simulink model "om_M4"  (R2016a)
settings: Solver=FixedStepAuto  StartTime=0.0  StopTime=10  FixedStep=0.0005  RelTol=1e-3
values from neighbouring files (symbols this model uses):
  Lm = 0.1271    [motor4_workspace.mat]    (also in motor_wrapper.m = obj.Lm; scim_verifier.m = obj.motor.getLm(); setMotorParams.m; stationary_class.m = obj.Lm)
  Lr = 0.2744    [motor4_workspace.mat]    (also in motor_wrapper.m = obj.Lr; scim_verifier.m = obj.motor.getLr(); setMotorParams.m; stationary_class.m = obj.Lr)
  Ls = 0.2744    [motor4_workspace.mat]    (also in motor_wrapper.m = obj.Ls; scim_verifier.m = obj.motor.getLs(); setMotorParams.m; stationary.m = Ls/10)
  M_ab02abc = [1  0  1; -0.5  0.866025403784  1; -0.5  -0.866025403784  1]    [motor4_workspace.mat]    (also in setMotorParams.m = inv(M_abc2ab0); workspaceSav.mat)
  M_abc2ab0 = [0.666666666667  -0.333333333333  -0.333333333333; 0  0.57735026919  -0.57735026919; 0.333333333333  0.333333333333  0.333333333333]    [motor4_workspace.mat]    (also in setMotorParams.m = [1, -0.5, -0.5; 0, sqrt(3)/2, -sqrt(3)/2;  0.5, 0.5, 0.5]; workspaceSav.mat)
  Rr = 1.009    [motor4_workspace.mat]    (also in motor_wrapper.m = obj.Rr; setMotorParams.m; stationary_class.m = obj.Rr; stationary_from_eq.m = obj.Rr)
  sig = (tox-fromx)/6    [gaussSpace.m]    (also in motor4_workspace.mat = 0.785452782217; setMotorParams.m = 0.785452782217; stationary_class.m = 1-Lm*Lm/Ls/Lr; torqueFinder.m = 0.785452782217)
libraries: powerlib_meascontrol x2, simulink x1, simulink_extras x1
settings Model: Creator=ebenera  LastModifiedBy=ebenera

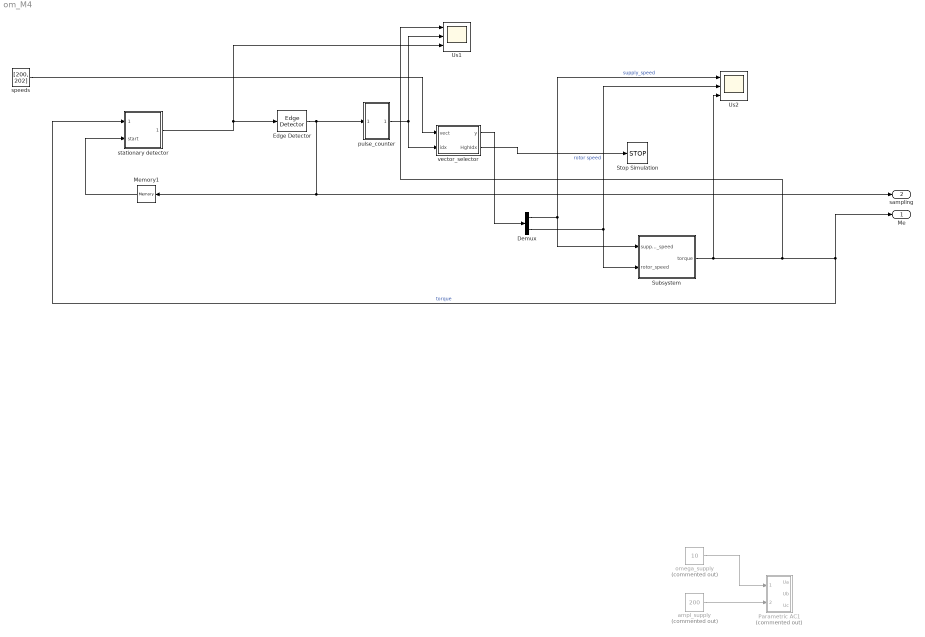
== system om_M4 ==
  Demux : Demux  Outputs=2
  Edge Detector : powerlib_meascontrol/Logic/Edge Detector  model=Rising  ic=0  Ts=0
  Memory1 : Memory  X0=1
  Parametric AC1 : Subsystem  Commented=on
  Stop Simulation : Stop
  Subsystem : Subsystem
  Us1 : Scope  NumInputPorts=3
  Us2 : Scope  NumInputPorts=3
  ampl_supply : Constant  Commented=on  Value=200
  omega_supply : Constant  Commented=on  Value=10
  pulse_counter : Subsystem
  speeds : Constant  Value=[200, 202]
  stationary detector : Subsystem
  vector_selector : MATLAB Function  TreatAsAtomicUnit=on
  Me : Outport
  sampling : Outport  Port=2
  wires:
  ampl_supply/1 -> Parametric AC1/2(Amp)
  omega_supply/1 -> Parametric AC1/1(Omega)
  speeds/1 -> vector_selector/1(vect)
  stationary detector/1(stable) -> Us1/3, Edge Detector/1
  vector_selector/2(HghIdx) -> Stop Simulation/1
  Subsystem/1(torque) -> Us2/3, Us1/1, stationary detector/1(state_var), Me/1  "torque"
  vector_selector/1(y) -> Demux/1
  Demux/2 -> Subsystem/2(rotor_speed), Us2/2  "rotor speed"
  Memory1/1 -> stationary detector/2(start)
  pulse_counter/1(Out1) -> vector_selector/2(idx), Us1/2
  Edge Detector/1 -> sampling/1, Memory1/1, pulse_counter/1(In1)
  Demux/1 -> Subsystem/1(supply_speed), Us2/1  "supply_speed"

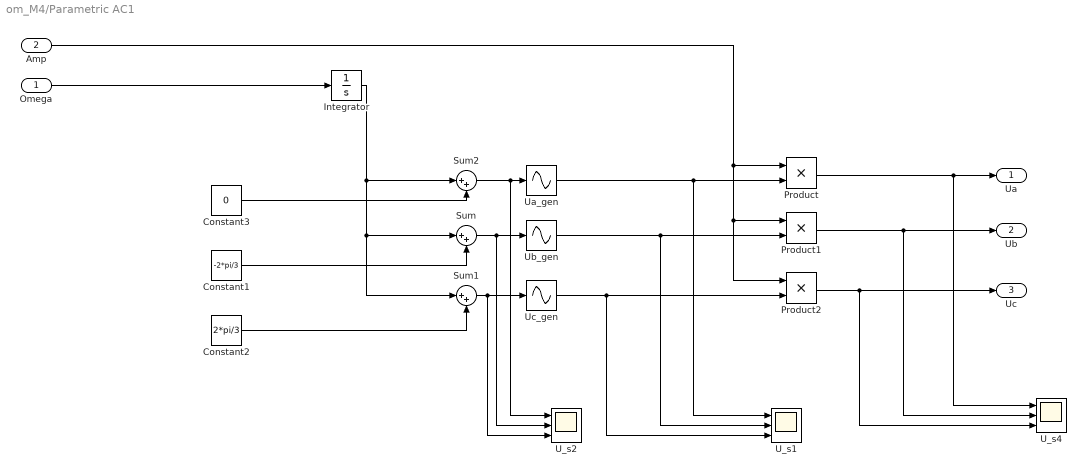
== system om_M4/Parametric AC1 ==
  Omega : Inport
  Amp : Inport  Port=2
  Constant1 : Constant  Value=-2*pi/3
  Constant2 : Constant  Value=2*pi/3
  Constant3 : Constant  Value=0
  Integrator : Integrator  WrapState=on
  Product : Product
  Product1 : Product
  Product2 : Product
  Sum : Sum  Inputs=|++
  Sum1 : Sum  Inputs=|++
  Sum2 : Sum  Inputs=|++
  U_s1 : Scope  NumInputPorts=3
  U_s2 : Scope  NumInputPorts=3
  U_s4 : Scope  NumInputPorts=3
  Ua_gen : Sin  TimeSource=Use external signal  SampleTime=0
  Ub_gen : Sin  TimeSource=Use external signal  SampleTime=0
  Uc_gen : Sin  TimeSource=Use external signal  SampleTime=0
  Ua : Outport
  Ub : Outport  Port=2
  Uc : Outport  Port=3
  wires:
  Sum/1 -> U_s2/2, Ub_gen/1
  Omega/1 -> Integrator/1
  Constant1/1 -> Sum/2
  Constant2/1 -> Sum1/2
  Sum1/1 -> U_s2/3, Uc_gen/1
  Sum2/1 -> U_s2/1, Ua_gen/1
  Constant3/1 -> Sum2/2
  Integrator/1 -> Sum2/1, Sum1/1, Sum/1
  Product/1 -> U_s4/1, Ua/1
  Product2/1 -> U_s4/3, Uc/1
  Product1/1 -> U_s4/2, Ub/1
  Amp/1 -> Product/1, Product1/1, Product2/1
  Ua_gen/1 -> U_s1/1, Product/2
  Uc_gen/1 -> U_s1/3, Product2/2
  Ub_gen/1 -> U_s1/2, Product1/2

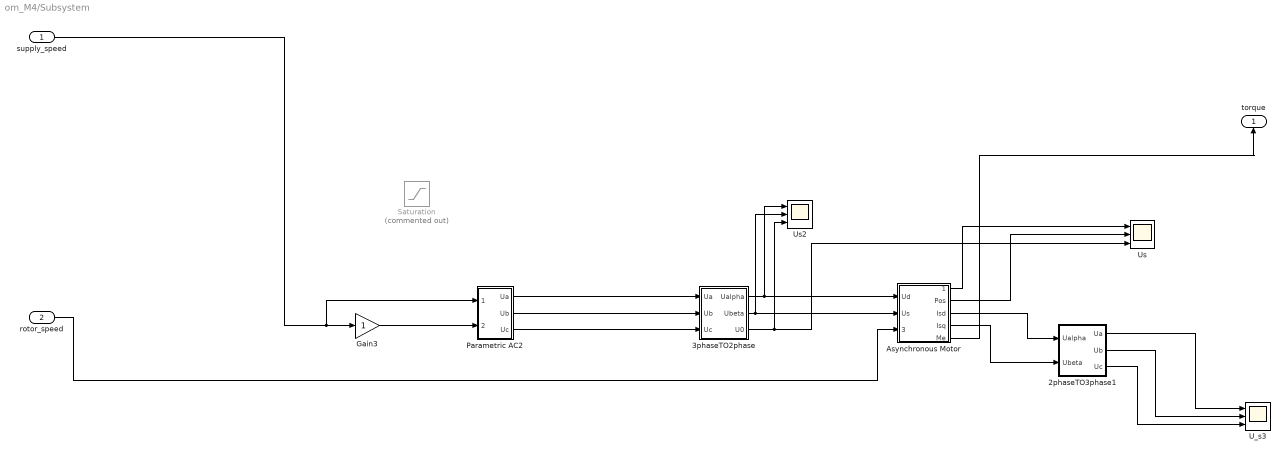
== system om_M4/Subsystem ==
  supply_speed : Inport
  rotor_speed : Inport  Port=2
  2phaseTO3phase1 : Subsystem
  "3phaseTO2phase " : Subsystem
  Asynchronous Motor : Subsystem
  Gain3 : Gain
  Parametric AC2 : Subsystem
  Saturation : Saturate  Commented=on  UpperLimit=300  LowerLimit=50
  U_s3 : Scope  NumInputPorts=3
  Us : Scope  NumInputPorts=3
  Us2 : Scope  NumInputPorts=3
  torque : Outport
  wires:
  "3phaseTO2phase "/1(Ualpha) -> Us2/1, Asynchronous Motor/1(Ud)
  "3phaseTO2phase "/2(Ubeta) -> Asynchronous Motor/2(Us), Us2/2
  Asynchronous Motor/4(Isq) -> 2phaseTO3phase1/2(Ubeta)
  Asynchronous Motor/3(Isd) -> 2phaseTO3phase1/1(Ualpha)
  2phaseTO3phase1/1(Ua) -> U_s3/1
  2phaseTO3phase1/2(Ub) -> U_s3/2
  2phaseTO3phase1/3(Uc) -> U_s3/3
  Parametric AC2/1(Ua) -> "3phaseTO2phase "/1(Ua)
  Parametric AC2/2(Ub) -> "3phaseTO2phase "/2(Ub)
  Parametric AC2/3(Uc) -> "3phaseTO2phase "/3(Uc)
  rotor_speed/1 -> Asynchronous Motor/3(OmegaIn)
  Asynchronous Motor/5(Me) -> torque/1
  Asynchronous Motor/1(Omega) -> Us/1
  Asynchronous Motor/2(Pos) -> Us/2
  "3phaseTO2phase "/3(U0) -> Us2/3, Us/3
  supply_speed/1 -> Gain3/1, Parametric AC2/1(Omega)
  Gain3/1 -> Parametric AC2/2(Amp)

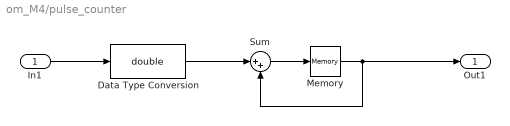
== system om_M4/pulse_counter ==
  In1 : Inport
  Data Type Conversion : DataTypeConversion  OutDataTypeStr=double  RndMeth=Ceiling
  Memory : Memory  X0=1
  Sum : Sum  Inputs=|++
  Out1 : Outport
  wires:
  Sum/1 -> Memory/1
  Memory/1 -> Sum/2, Out1/1
  In1/1 -> Data Type Conversion/1
  Data Type Conversion/1 -> Sum/1

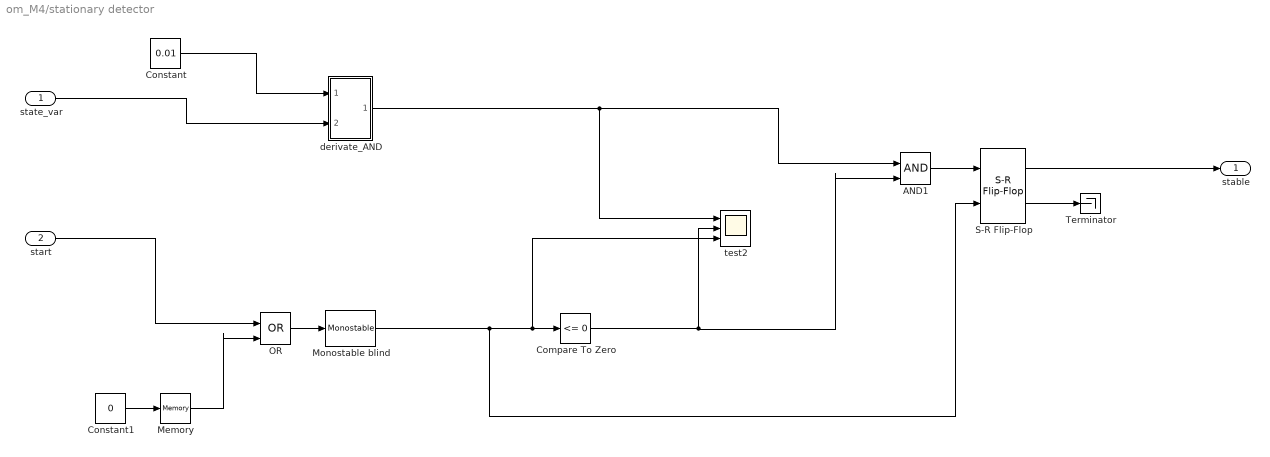
== system om_M4/stationary detector ==
  state_var : Inport
  start : Inport  Port=2
  AND1 : Logic  IconShape=distinctive  AllPortsSameDT=off  OutDataTypeStr=boolean
  Compare To Zero : simulink/Logic and Bit Operations/Compare To Zero  relop=<=  OutDataTypeStr=boolean
  Constant : Constant  Value=0.01
  Constant1 : Constant  Value=0
  Memory : Memory  X0=1
  Monostable blind : powerlib_meascontrol/Logic/Monostable  EdgeDetect=Either  PulseDuration=0.1  ic=0  Ts=0
  OR : Logic  Operator=OR  IconShape=distinctive  AllPortsSameDT=off  OutDataTypeStr=boolean
  S-R Flip-Flop : simulink_extras/Flip Flops/S-R Flip-Flop  initial_condition=0
  Terminator : Terminator
  derivate_AND : Subsystem
  test2 : Scope  NumInputPorts=3
  stable : Outport
  wires:
  Compare To Zero/1 -> AND1/2, test2/2
  S-R Flip-Flop/1 -> stable/1
  AND1/1 -> S-R Flip-Flop/1
  derivate_AND/1(Out1) -> AND1/1, test2/1
  Constant/1 -> derivate_AND/1(In1)
  state_var/1 -> derivate_AND/2(In2)
  Monostable blind/1 -> S-R Flip-Flop/2, test2/3, Compare To Zero/1
  Constant1/1 -> Memory/1
  Memory/1 -> OR/2
  start/1 -> OR/1
  OR/1 -> Monostable blind/1
  S-R Flip-Flop/2 -> Terminator/1

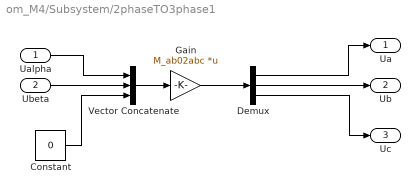
== system om_M4/Subsystem/2phaseTO3phase1 ==
  Ualpha : Inport
  Ubeta : Inport  Port=2
  Constant : Constant  Value=0
  Demux : Demux  Outputs=3
  Gain : Gain  Gain=M_ab02abc  Multiplication=Matrix(K*u)
  Vector Concatenate : Concatenate  NumInputs=3
  Ua : Outport
  Ub : Outport  Port=2
  Uc : Outport  Port=3
  wires:
  Vector Concatenate/1 -> Gain/1
  Ualpha/1 -> Vector Concatenate/1
  Demux/3 -> Uc/1
  Gain/1 -> Demux/1
  Constant/1 -> Vector Concatenate/3
  Ubeta/1 -> Vector Concatenate/2
  Demux/1 -> Ua/1
  Demux/2 -> Ub/1

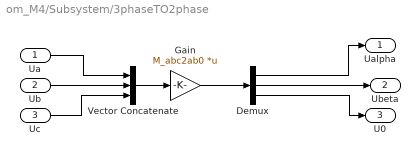
== system om_M4/Subsystem/3phaseTO2phase  ==
  Ua : Inport
  Ub : Inport  Port=2
  Uc : Inport  Port=3
  Demux : Demux  Outputs=3
  Gain : Gain  Gain=M_abc2ab0  Multiplication=Matrix(K*u)
  Vector Concatenate : Concatenate  NumInputs=3
  Ualpha : Outport
  Ubeta : Outport  Port=2
  U0 : Outport  Port=3
  wires:
  Vector Concatenate/1 -> Gain/1
  Ua/1 -> Vector Concatenate/1
  Demux/3 -> U0/1
  Gain/1 -> Demux/1
  Uc/1 -> Vector Concatenate/3
  Ub/1 -> Vector Concatenate/2
  Demux/1 -> Ualpha/1
  Demux/2 -> Ubeta/1

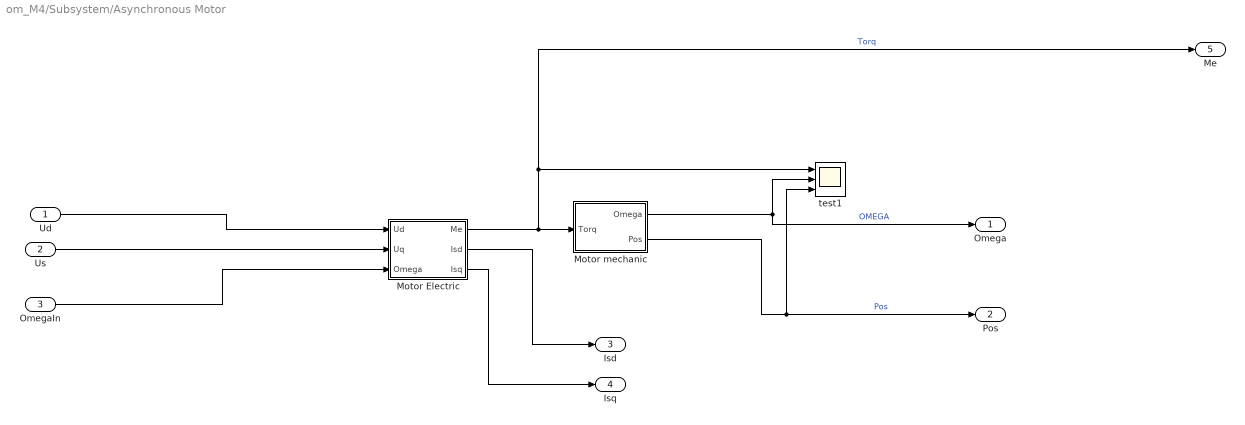
== system om_M4/Subsystem/Asynchronous Motor ==
  Ud : Inport
  Us : Inport  Port=2
  OmegaIn : Inport  Port=3
  Motor Electric : Subsystem
  Motor mechanic : Subsystem
  test1 : Scope  NumInputPorts=3
  Omega : Outport
  Pos : Outport  Port=2
  Isd : Outport  Port=3
  Isq : Outport  Port=4
  Me : Outport  Port=5
  wires:
  Motor mechanic/2(Pos) -> test1/3, Pos/1  "Pos"
  Motor mechanic/1(Omega) -> test1/2, Omega/1  "OMEGA"
  Motor Electric/1(Me) -> Me/1, test1/1, Motor mechanic/1("Torq ")  "Torq"
  Motor Electric/2(Isd) -> Isd/1
  Motor Electric/3(Isq) -> Isq/1
  Us/1 -> Motor Electric/2(Uq)
  Ud/1 -> Motor Electric/1(Ud)
  OmegaIn/1 -> Motor Electric/3(Omega)

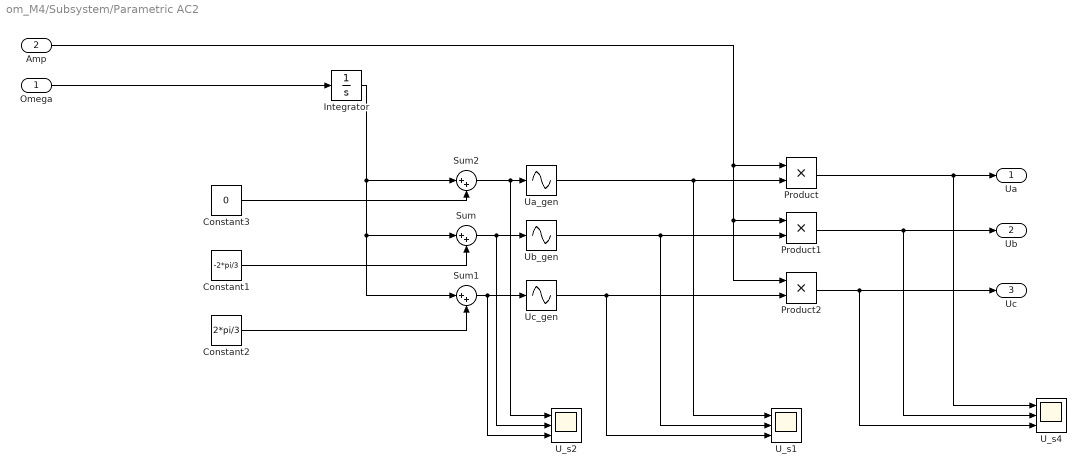
== system om_M4/Subsystem/Parametric AC2 ==
  Omega : Inport
  Amp : Inport  Port=2
  Constant1 : Constant  Value=-2*pi/3
  Constant2 : Constant  Value=2*pi/3
  Constant3 : Constant  Value=0
  Integrator : Integrator  WrapState=on
  Product : Product
  Product1 : Product
  Product2 : Product
  Sum : Sum  Inputs=|++
  Sum1 : Sum  Inputs=|++
  Sum2 : Sum  Inputs=|++
  U_s1 : Scope  NumInputPorts=3
  U_s2 : Scope  NumInputPorts=3
  U_s4 : Scope  NumInputPorts=3
  Ua_gen : Sin  TimeSource=Use external signal  SampleTime=0
  Ub_gen : Sin  TimeSource=Use external signal  SampleTime=0
  Uc_gen : Sin  TimeSource=Use external signal  SampleTime=0
  Ua : Outport
  Ub : Outport  Port=2
  Uc : Outport  Port=3
  wires:
  Sum/1 -> U_s2/2, Ub_gen/1
  Omega/1 -> Integrator/1
  Constant1/1 -> Sum/2
  Constant2/1 -> Sum1/2
  Sum1/1 -> U_s2/3, Uc_gen/1
  Sum2/1 -> U_s2/1, Ua_gen/1
  Constant3/1 -> Sum2/2
  Integrator/1 -> Sum2/1, Sum1/1, Sum/1
  Product/1 -> U_s4/1, Ua/1
  Product2/1 -> U_s4/3, Uc/1
  Product1/1 -> U_s4/2, Ub/1
  Amp/1 -> Product/1, Product1/1, Product2/1
  Ua_gen/1 -> U_s1/1, Product/2
  Uc_gen/1 -> U_s1/3, Product2/2
  Ub_gen/1 -> U_s1/2, Product1/2

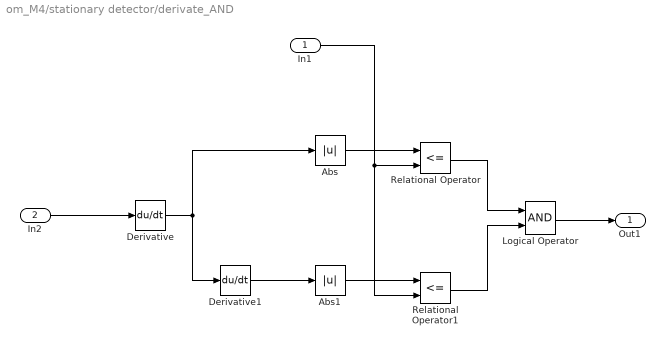
== system om_M4/stationary detector/derivate_AND ==
  In1 : Inport
  In2 : Inport  Port=2
  Abs : Abs
  Abs1 : Abs
  Derivative : Derivative
  Derivative1 : Derivative
  Logical Operator : Logic  AllPortsSameDT=off  OutDataTypeStr=boolean
  Relational Operator : RelationalOperator  Operator=<=  OutDataTypeStr=boolean
  Relational Operator1 : RelationalOperator  Operator=<=  OutDataTypeStr=boolean
  Out1 : Outport
  wires:
  In2/1 -> Derivative/1
  Derivative/1 -> Abs/1, Derivative1/1
  In1/1 -> Relational Operator1/2, Relational Operator/2
  Relational Operator/1 -> Logical Operator/1
  Relational Operator1/1 -> Logical Operator/2
  Abs/1 -> Relational Operator/1
  Abs1/1 -> Relational Operator1/1
  Derivative1/1 -> Abs1/1
  Logical Operator/1 -> Out1/1

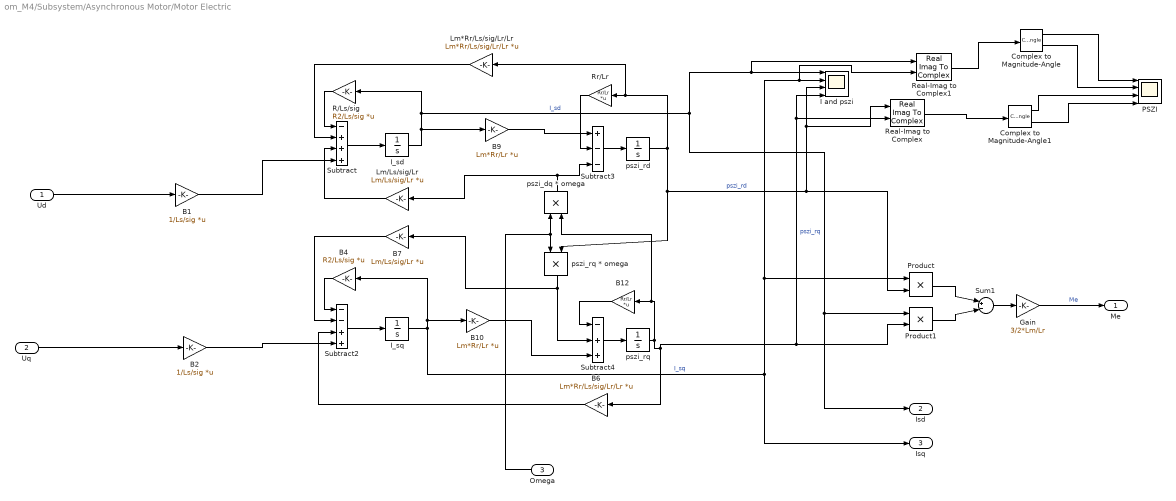
== system om_M4/Subsystem/Asynchronous Motor/Motor Electric ==
  Ud : Inport
  Uq : Inport  Port=2
  Omega : Inport  Port=3
  B1 : Gain  Gain=1/Ls/sig  Multiplication=Matrix(K*u)
  B10 : Gain  Gain=Lm*Rr/Lr  Multiplication=Matrix(K*u)
  B12 : Gain  Gain=Rr/Lr  Multiplication=Matrix(K*u)
  B2 : Gain  Gain=1/Ls/sig  Multiplication=Matrix(K*u)
  B4 : Gain  Gain=R2/Ls/sig  Multiplication=Matrix(K*u)
  B6 : Gain  Gain=Lm*Rr/Ls/sig/Lr/Lr  Multiplication=Matrix(K*u)
  B7 : Gain  Gain=Lm/Ls/sig/Lr  Multiplication=Matrix(K*u)
  B9 : Gain  Gain=Lm*Rr/Lr  Multiplication=Matrix(K*u)
  Complex to Magnitude-Angle : ComplexToMagnitudeAngle
  Complex to Magnitude-Angle1 : ComplexToMagnitudeAngle
  Gain : Gain  Gain=3/2*Lm/Lr
  I and pszi : Scope  NumInputPorts=4
  I_sd : Integrator
  I_sq : Integrator
  Lm*Rr/Ls/sig/Lr/Lr : Gain  Gain=Lm*Rr/Ls/sig/Lr/Lr  Multiplication=Matrix(K*u)
  Lm/Ls/sig/Lr : Gain  Gain=Lm/Ls/sig/Lr  Multiplication=Matrix(K*u)
  PSZI : Scope  NumInputPorts=4
  Product : Product
  Product1 : Product
  R/Ls/sig : Gain  Gain=R2/Ls/sig  Multiplication=Matrix(K*u)
  Real-Imag to Complex : RealImagToComplex
  Real-Imag to Complex1 : RealImagToComplex
  Rr/Lr : Gain  Gain=Rr/Lr  Multiplication=Matrix(K*u)
  Subtract : Sum  Inputs=-+++
  Subtract2 : Sum  Inputs=--++
  Subtract3 : Sum  Inputs=+--
  Subtract4 : Sum  Inputs=-++
  Sum1 : Sum  Inputs=|+-|
  pszi_dq * omega : Product
  pszi_rd : Integrator
  "pszi_rq " : Integrator
  pszi_rq * omega : Product
  Me : Outport
  Isd : Outport  Port=2
  Isq : Outport  Port=3
  wires:
  pszi_rq * omega/1 -> Subtract4/2, B7/1
  Subtract/1 -> I_sd/1
  B12/1 -> Subtract4/1
  Product1/1 -> Sum1/2
  Lm*Rr/Ls/sig/Lr/Lr/1 -> Subtract/2
  Product/1 -> Sum1/1
  I_sq/1 -> Isq/1, Real-Imag to Complex1/2, I and pszi/2, Product/1, B10/1, B4/1  "I_sq"
  I_sd/1 -> B9/1, Isd/1, Product1/1, Real-Imag to Complex1/1, I and pszi/1, R/Ls/sig/1  "I_sd"
  Sum1/1 -> Gain/1
  R/Ls/sig/1 -> Subtract/1
  B6/1 -> Subtract2/3
  B4/1 -> Subtract2/1
  pszi_dq * omega/1 -> Subtract3/3, Lm/Ls/sig/Lr/1
  Omega/1 -> pszi_rq * omega/1, pszi_dq * omega/1
  B9/1 -> Subtract3/1
  Rr/Lr/1 -> Subtract3/2
  pszi_rd/1 -> Real-Imag to Complex/1, I and pszi/3, Product/2, pszi_rq * omega/2, Lm*Rr/Ls/sig/Lr/Lr/1, Rr/Lr/1  "pszi_rd"
  Lm/Ls/sig/Lr/1 -> Subtract/3
  "pszi_rq "/1 -> pszi_dq * omega/2, B12/1, Real-Imag to Complex/2, I and pszi/4, Product1/2, B6/1  "pszi_rq"
  B7/1 -> Subtract2/2
  Gain/1 -> Me/1  "Me"
  B10/1 -> Subtract4/3
  Subtract4/1 -> "pszi_rq "/1
  Subtract2/1 -> I_sq/1
  Subtract3/1 -> pszi_rd/1
  Uq/1 -> B2/1
  Ud/1 -> B1/1
  B1/1 -> Subtract/4
  B2/1 -> Subtract2/4
  Real-Imag to Complex1/1 -> Complex to Magnitude-Angle/1
  Complex to Magnitude-Angle/1 -> PSZI/1
  Complex to Magnitude-Angle/2 -> PSZI/2
  Real-Imag to Complex/1 -> Complex to Magnitude-Angle1/1
  Complex to Magnitude-Angle1/1 -> PSZI/3
  Complex to Magnitude-Angle1/2 -> PSZI/4

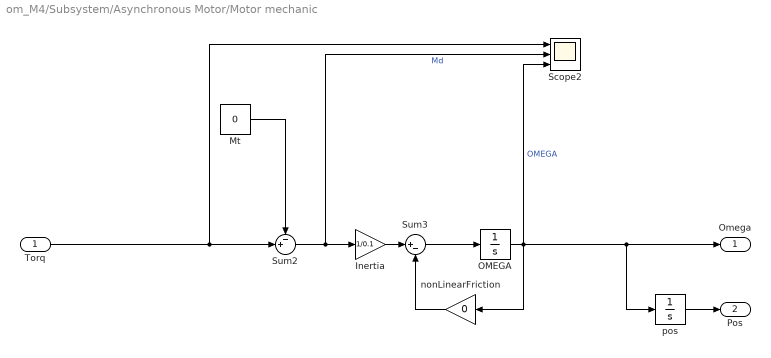
== system om_M4/Subsystem/Asynchronous Motor/Motor mechanic ==
  "Torq " : Inport
  Inertia : Gain  Gain=1/0.1
  Mt : Constant  Value=0
  OMEGA : Integrator
  Scope2 : Scope  NumInputPorts=3
  Sum2 : Sum  Inputs=-+|
  Sum3 : Sum  Inputs=|+-
  nonLinearFriction : Gain  Gain=0
  pos : Integrator  WrapState=on
  Omega : Outport
  Pos : Outport  Port=2
  wires:
  "Torq "/1 -> Scope2/1, Sum2/2
  OMEGA/1 -> Scope2/3, pos/1, Omega/1, nonLinearFriction/1  "OMEGA"
  Sum3/1 -> OMEGA/1
  Sum2/1 -> Inertia/1, Scope2/2  "Md"
  Mt/1 -> Sum2/1
  nonLinearFriction/1 -> Sum3/2
  Inertia/1 -> Sum3/1
  pos/1 -> Pos/1

== matlab function om_M4/vector_selector ==
  data: vect input; y output; idx input; HghIdx output
function [y, HghIdx] = fcn(vect, idx)
    if(idx>length(vect(1,:)))
        HghIdx = 1;
        y = [0; 0];
    else
        HghIdx = 0;
        y = vect(:,idx);
    end
end
